simulink model "estimador_discreto"  (R2014b)
settings: Solver=ode23t  StartTime=0.0  StopTime=50e-3  RelTol=1e-3
model workspace (MAT data in the model file):
  kh = Simulink.Parameter
  kh.Value = 0.05
  kh.DataType = 'auto'
  C1 = Simulink.Parameter
  C1.Value = 1e-06
  C1.DataType = 'auto'
  R1 = Simulink.Parameter
  R1.Value = 25000
  R1.DataType = 'auto'
  RL = Simulink.Parameter
  RL.Value = 0.2
  RL.DataType = 'auto'
  Lyo = Simulink.Parameter
  Lyo.Value = 0.01621
  Lyo.DataType = 'auto'
settings Model: Creator=Javi  LastModifiedBy=Javi

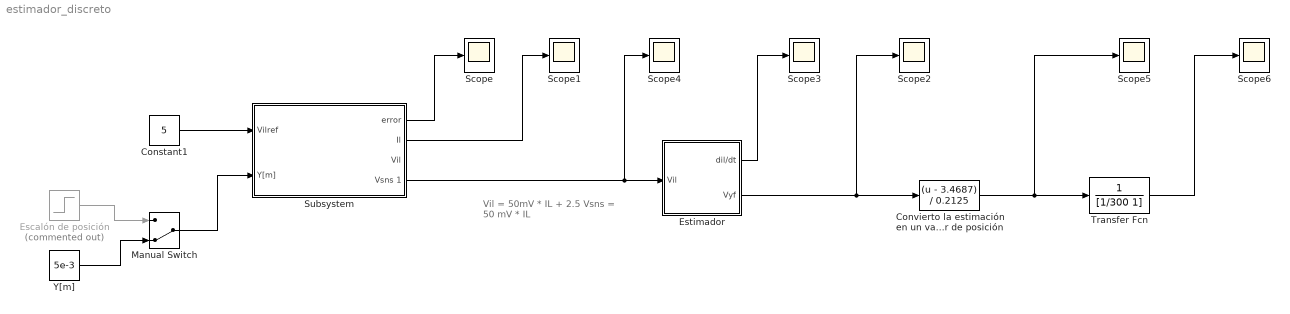
== system estimador_discreto ==
  note: Vil = 50mV * IL + 2.5
      | Vsns = 50 mV * IL
  Constant1 : Constant  Value=5  SampleTime=1/50000
  "Convierto la estimación en un valor de posición " : Fcn  Expr=(u - 3.4687) / 0.2125
  "Escalón de posición " : Step  Commented=on  Time=10e-3  Before=2e-3  After=5e-3  SampleTime=0
  "Estimador " : Subsystem
  Manual Switch : ManualSwitch  CurrentSetting=0
  Scope{,1..6} (7 alike) : Scope
      Scope settings: TimeRange=0.015  YMin=2.4  YMax=3.1
      Scope1 settings: TimeRange=0.035  YMin=0  YMax=7
      Scope2 settings: TimeRange=0.015  YMin=3.45  YMax=3.75  SaveName=ScopeData2
      Scope3 settings: TimeRange=0.035  YMin=2.35  YMax=2.65  SaveName=ScopeData3
      Scope4 settings: TimeRange=0.035  YMin=0  YMax=0.7000000000000001  SaveName=Corriente  SampleInput=on  SampleTime=1/50000
      Scope5 settings: TimeRange=0.015  YMin=3.45  YMax=3.75  SaveName=ScopeData6
      Scope6 settings: TimeRange=0.015  YMin=3.45  YMax=3.75  SaveName=ScopeData4
  Subsystem : Subsystem
  Transfer Fcn : TransferFcn  Numerator=1  Denominator=[1/300 1]
  Y[m] : Constant  Value=5e-3
  wires:
  Subsystem/1("error ") -> Scope/1
  Subsystem/2("Il ") -> Scope1/1
  "Estimador "/1(dil/dt) -> Scope3/1
  "Estimador "/2(Vyf) -> Scope2/1, "Convierto la estimación en un valor de posición "/1
  Constant1/1 -> Subsystem/1("Vilref ")
  Y[m]/1 -> Manual Switch/2
  "Escalón de posición "/1 -> Manual Switch/1
  Manual Switch/1 -> Subsystem/2("Y[m] ")
  Subsystem/4(Vsns 1) -> Scope4/1, "Estimador "/1(Vil)
  Transfer Fcn/1 -> Scope6/1
  "Convierto la estimación en un valor de posición "/1 -> Transfer Fcn/1, Scope5/1

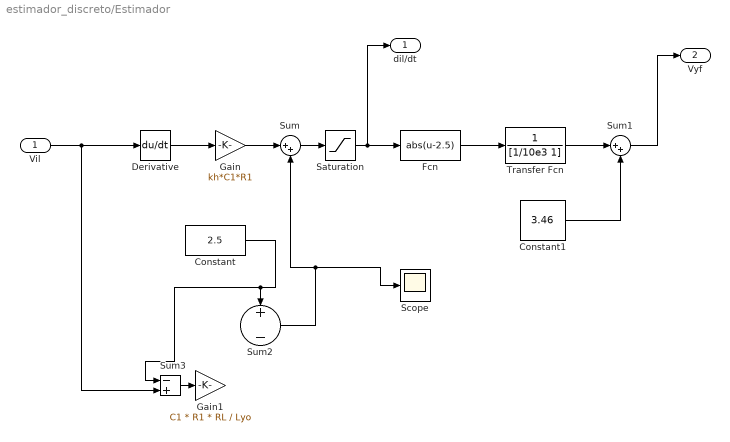
== system estimador_discreto/Estimador  ==
  Vil : Inport
  Constant : Constant  Value=2.5
  Constant1 : Constant  Value=3.46
  Derivative : Derivative
  Fcn : Fcn  Expr=abs(u-2.5)
  Gain : Gain  Gain=kh*C1*R1  SampleTime=1/50000
  Gain1 : Gain  Gain=C1 * R1 * RL / Lyo
  Saturation : Saturate  UpperLimit=5  LowerLimit=0
  Scope : Scope
      settings: SaveName=ScopeData5
  Sum : Sum  Inputs=|++
  Sum1 : Sum  Inputs=|++
  Sum2 : Sum  Inputs=+-
  Sum3 : Sum  Inputs=-+
  Transfer Fcn : TransferFcn  Denominator=[1/10e3 1]
  dil/dt : Outport
  Vyf : Outport  Port=2
  wires:
  Vil/1 -> Derivative/1, Sum3/2
  Derivative/1 -> Gain/1
  Saturation/1 -> Fcn/1, dil/dt/1
  Gain/1 -> Sum/1
  Sum/1 -> Saturation/1
  Constant/1 -> Sum3/1, Sum2/1
  Fcn/1 -> Transfer Fcn/1
  Sum1/1 -> Vyf/1
  Transfer Fcn/1 -> Sum1/1
  Sum2/1 -> Scope/1, Sum/2
  Sum3/1 -> Gain1/1
  Constant1/1 -> Sum1/2

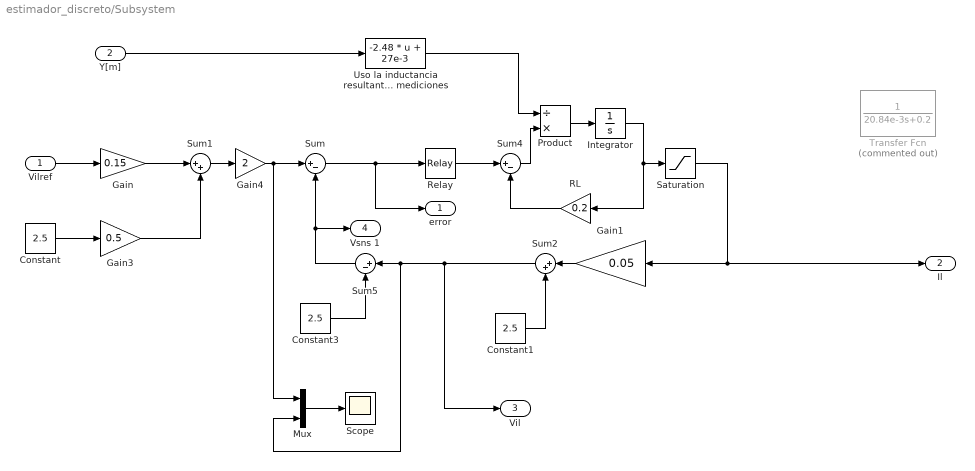
== system estimador_discreto/Subsystem ==
  "Vilref " : Inport
  "Y[m] " : Inport  Port=2
  Constant : Constant  Value=2.5
  Constant1 : Constant  Value=2.5
  Constant3 : Constant  Value=2.5
  Gain : Gain  Gain=0.15
  Gain1 : Gain  Gain=0.05
  Gain3 : Gain  Gain=0.5
  Gain4 : Gain  Gain=2
  Integrator : Integrator
  Mux : Mux  Inputs=2
  Product : Product  Inputs=/*
  RL : Gain  Gain=0.2
  Relay : Relay  OnSwitchValue=2.5125  OffSwitchValue=2.4875  OnOutputValue=24  OffOutputValue=-24
  Saturation : Saturate  UpperLimit=40  LowerLimit=0  SampleTime=1/50000
  Scope : Scope
      settings: SaveName=ScopeData2
  Sum : Sum  Inputs=|+-
  Sum1 : Sum  Inputs=|++
  Sum2 : Sum  Inputs=|++
  Sum4 : Sum  Inputs=|+-
  Sum5 : Sum  Inputs=|+-
  Transfer Fcn : TransferFcn  Commented=on  Denominator=[20.84e-3 0.2]
  "Uso la inductancia resultante de las mediciones " : Fcn  Expr=-2.48 * u + 27e-3
  "error " : Outport
  "Il " : Outport  Port=2
  "Vil " : Outport  Port=3
  Vsns 1 : Outport  Port=4
  wires:
  Sum1/1 -> Gain4/1
  Gain4/1 -> Sum/1, Mux/1
  Gain3/1 -> Sum1/2
  Gain/1 -> Sum1/1
  Saturation/1 -> "Il "/1, Gain1/1
  Constant/1 -> Gain3/1
  "Vilref "/1 -> Gain/1
  Mux/1 -> Scope/1
  Constant1/1 -> Sum2/2
  Gain1/1 -> Sum2/1
  Sum2/1 -> "Vil "/1, Sum5/1, Mux/2
  Sum/1 -> Relay/1, "error "/1
  Relay/1 -> Sum4/1
  Integrator/1 -> RL/1, Saturation/1
  Product/1 -> Integrator/1
  Sum4/1 -> Product/2
  "Y[m] "/1 -> "Uso la inductancia resultante de las mediciones "/1
  "Uso la inductancia resultante de las mediciones "/1 -> Product/1
  Constant3/1 -> Sum5/2
  Sum5/1 -> Vsns 1/1, Sum/2
  RL/1 -> Sum4/2
